simulink model "TehnikaA"  (R2016a)
settings: Solver=VariableStepAuto  StartTime=0.0  StopTime=10.0  MaxStep=1e-3  RelTol=1e-3
InitFcn:
  | parametriAM
values from neighbouring files (symbols this model uses):
  Imrn = 7.4    [parametriAM.m]
  In = 12.7    [parametriAM.m]
  Ls = 0.05315    [parametriAM.m]    (also in podatki.m = 0.2449)
  Lst = sigma*Ls    (= 0.00742111947319)    [parametriAM.m]
  Un = 216    [parametriAM.m]
libraries: simulink x3
settings Model: Creator=Mitja1  LastModifiedBy=Mitja1

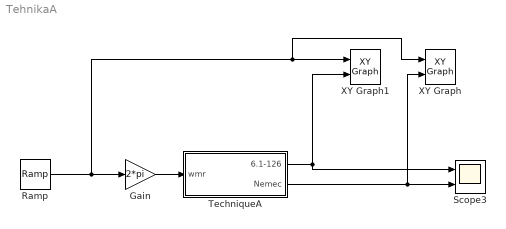
== system TehnikaA ==
  Gain : Gain  Gain=2*pi
  Ramp : simulink/Sources/Ramp  slope=40  start=0  X0=0
  Scope3 : Scope  NumInputPorts=2
  TechniqueA : Subsystem
  XY Graph : simulink/Sinks/XY Graph  xmin=0  xmax=400  ymin=0  ymax=15  st=-1
  XY Graph1 : simulink/Sinks/XY Graph  xmin=0  xmax=400  ymin=0  ymax=15  st=-1
  wires:
  TechniqueA/1(6.1-126) -> Scope3/1, XY Graph1/2
  TechniqueA/2(Nemec) -> Scope3/2, XY Graph/2
  Ramp/1 -> XY Graph1/1, XY Graph/1, Gain/1
  Gain/1 -> TechniqueA/1(wmr)

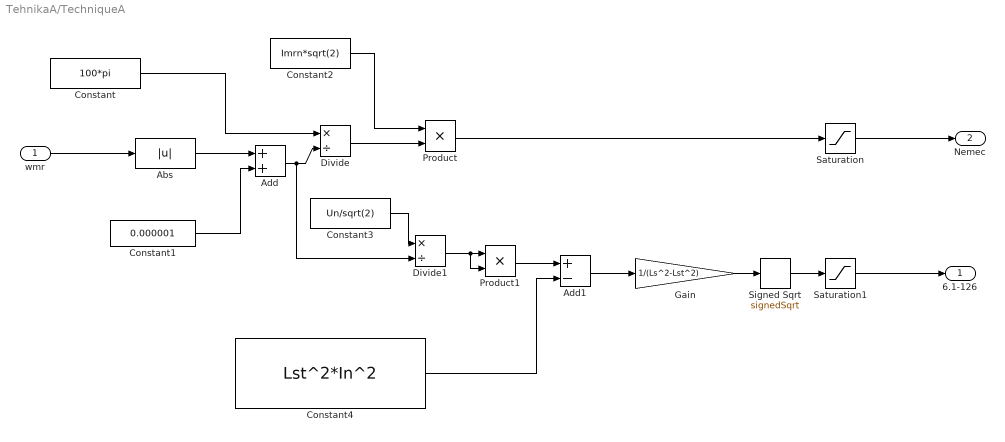
== system TehnikaA/TechniqueA ==
  wmr : Inport
  Abs : Abs
  Add : Sum
  Add1 : Sum  Inputs=+-
  Constant : Constant  Value=100*pi
  Constant1 : Constant  Value=0.000001
  Constant2 : Constant  Value=Imrn*sqrt(2)
  Constant3 : Constant  Value=Un/sqrt(2)
  Constant4 : Constant  Value=Lst^2*In^2
  Divide : Product  Inputs=*/
  Divide1 : Product  Inputs=*/
  Gain : Gain  Gain=1/(Ls^2-Lst^2)
  Product : Product
  Product1 : Product
  Saturation : Saturate  UpperLimit=+Imrn*sqrt(2)  LowerLimit=0
  Saturation1 : Saturate  UpperLimit=+Imrn*sqrt(2)  LowerLimit=0
  Signed Sqrt : Sqrt  Operator=signedSqrt  SaturateOnIntegerOverflow=on
  6.1-126 : Outport
  Nemec : Outport  Port=2
  wires:
  Constant2/1 -> Product/1
  wmr/1 -> Abs/1
  Divide/1 -> Product/2
  Product/1 -> Saturation/1
  Constant/1 -> Divide/1
  Add/1 -> Divide1/2, Divide/2
  Abs/1 -> Add/1
  Constant1/1 -> Add/2
  Saturation/1 -> Nemec/1
  Constant3/1 -> Divide1/1
  Divide1/1 -> Product1/2, Product1/1
  Product1/1 -> Add1/1
  Constant4/1 -> Add1/2
  Saturation1/1 -> 6.1-126/1
  Add1/1 -> Gain/1
  Gain/1 -> Signed Sqrt/1
  Signed Sqrt/1 -> Saturation1/1
